simulink model "IEEE9_case"  (R2024b)
settings: Solver=FixedStepAuto  StartTime=0  StopTime=5  FixedStep=1e-7  RelTol=1e-3
values from neighbouring files (symbols this model uses):
  SG_D_1_D = 0.01056    [IEEE9_case_parameters.m]    (also in case1_parameters.m; case2_parameters.m; case3_parameters.m; case4_parameters.m)
  SG_D_1_EnableSaturation = 0    [IEEE9_case_parameters.m]    (also in case1_parameters.m; case2_parameters.m; case3_parameters.m; case4_parameters.m)
  SG_D_1_f0 = 60    [IEEE9_case_parameters.m]    (also in case1_parameters.m; case2_parameters.m; case3_parameters.m; case4_parameters.m)
  SG_D_1_H = 7.5    [IEEE9_case_parameters.m]    (also in case1_parameters.m; case2_parameters.m; case3_parameters.m; case4_parameters.m)
  SG_D_1_K_A = 20    [IEEE9_case_parameters.m]    (also in case1_parameters.m; case2_parameters.m; case3_parameters.m; case4_parameters.m)
  SG_D_1_K_E = 1.000000e+1    (= 10)    [IEEE9_case_parameters.m]    (also in case1_parameters.m; case2_parameters.m; case3_parameters.m; case4_parameters.m)
  SG_D_1_K_F = 2.363    [IEEE9_case_parameters.m]    (also in case1_parameters.m; case2_parameters.m; case3_parameters.m; case4_parameters.m)
  SG_D_1_K_s = 0.5    [IEEE9_case_parameters.m]    (also in case1_parameters.m = 5; case2_parameters.m = 5; case3_parameters.m = 5; case4_parameters.m = 5)
  SG_D_1_R_a = 0.001088    [IEEE9_case_parameters.m]    (also in case1_parameters.m; case2_parameters.m; case3_parameters.m; case4_parameters.m)
  SG_D_1_S_A = 1    [IEEE9_case_parameters.m]    (also in case1_parameters.m; case2_parameters.m; case3_parameters.m; case4_parameters.m)
  SG_D_1_S_B = 0.103    [IEEE9_case_parameters.m]    (also in case1_parameters.m; case2_parameters.m; case3_parameters.m; case4_parameters.m)
  SG_D_1_S_N = 10.659857    [IEEE9_case_parameters.m]    (also in case1_parameters.m; case2_parameters.m; case3_parameters.m; case4_parameters.m)
  SG_D_1_SpeedPara = 200    [IEEE9_case_parameters.m]    (also in case1_parameters.m; case2_parameters.m; case3_parameters.m; case4_parameters.m)
  SG_D_1_T_0 = 0.720173    [IEEE9_case_parameters.m]    (also in case1_parameters.m = 0.755522; case2_parameters.m = 0.808931; case3_parameters.m = 0.869402; case4_parameters.m = 0.729316)
  SG_D_1_T_1 = 0.3    [IEEE9_case_parameters.m]    (also in case1_parameters.m; case2_parameters.m; case3_parameters.m; case4_parameters.m)
  SG_D_1_T_2 = 0.05    [IEEE9_case_parameters.m]    (also in case1_parameters.m; case2_parameters.m; case3_parameters.m; case4_parameters.m)
  SG_D_1_T_3 = 0.02    [IEEE9_case_parameters.m]    (also in case1_parameters.m; case2_parameters.m; case3_parameters.m; case4_parameters.m)
  SG_D_1_T_4 = 0.005    [IEEE9_case_parameters.m]    (also in case1_parameters.m; case2_parameters.m; case3_parameters.m; case4_parameters.m)
  SG_D_1_T_A = 0.02    [IEEE9_case_parameters.m]    (also in case1_parameters.m; case2_parameters.m; case3_parameters.m; case4_parameters.m)
  SG_D_1_T_dd = 8.000000e+0    (= 8)    [IEEE9_case_parameters.m]    (also in case1_parameters.m; case2_parameters.m; case3_parameters.m; case4_parameters.m)
  SG_D_1_T_ddd = 0.04    [IEEE9_case_parameters.m]    (also in case1_parameters.m; case2_parameters.m; case3_parameters.m; case4_parameters.m)
  SG_D_1_T_E = 0.314    [IEEE9_case_parameters.m]    (also in case1_parameters.m; case2_parameters.m; case3_parameters.m; case4_parameters.m)
  SG_D_1_T_F = 0.35    [IEEE9_case_parameters.m]    (also in case1_parameters.m; case2_parameters.m; case3_parameters.m; case4_parameters.m)
  SG_D_1_T_qd = 0.8    [IEEE9_case_parameters.m]    (also in case1_parameters.m; case2_parameters.m; case3_parameters.m; case4_parameters.m)
  SG_D_1_T_qdd = 0.02    [IEEE9_case_parameters.m]    (also in case1_parameters.m; case2_parameters.m; case3_parameters.m; case4_parameters.m)
  SG_D_1_T_speed = 0.1    [IEEE9_case_parameters.m]    (also in case1_parameters.m = 200; case2_parameters.m = 200; case3_parameters.m = 200; case4_parameters.m = 200)
  SG_D_1_T_w = 0.5    [IEEE9_case_parameters.m]    (also in case1_parameters.m; case2_parameters.m; case3_parameters.m; case4_parameters.m)
  SG_D_1_V_ref = 1.990276    [IEEE9_case_parameters.m]    (also in case1_parameters.m = 2.042296; case2_parameters.m = 2.051388; case3_parameters.m = 2.089584; case4_parameters.m = 2.01845)
  SG_D_1_w_ref = 376.991118    [IEEE9_case_parameters.m]    (also in case1_parameters.m; case2_parameters.m; case3_parameters.m; case4_parameters.m)
  SG_D_1_wb = 6.000000e+1    (= 60)    [IEEE9_case_parameters.m]    (also in case1_parameters.m; case2_parameters.m; case3_parameters.m; case4_parameters.m)
  SG_D_1_x_d = 1.9    [IEEE9_case_parameters.m]    (also in case1_parameters.m; case2_parameters.m; case3_parameters.m; case4_parameters.m)
  SG_D_1_x_dd = 0.302    [IEEE9_case_parameters.m]    (also in case1_parameters.m; case2_parameters.m; case3_parameters.m; case4_parameters.m)
  SG_D_1_x_ddd = 0.204    [IEEE9_case_parameters.m]    (also in case1_parameters.m; case2_parameters.m; case3_parameters.m; case4_parameters.m)
  SG_D_1_x_l = 0.05    [IEEE9_case_parameters.m]    (also in case1_parameters.m; case2_parameters.m; case3_parameters.m; case4_parameters.m)
  SG_D_1_x_q = 1.3    [IEEE9_case_parameters.m]    (also in case1_parameters.m; case2_parameters.m; case3_parameters.m; case4_parameters.m)
  SG_D_1_x_qd = 0.5    [IEEE9_case_parameters.m]    (also in case1_parameters.m; case2_parameters.m; case3_parameters.m; case4_parameters.m)
  SG_D_1_x_qdd = 0.3    [IEEE9_case_parameters.m]    (also in case1_parameters.m; case2_parameters.m; case3_parameters.m; case4_parameters.m)
  SG_D_2_D = 0.02    [IEEE9_case_parameters.m]    (also in case1_parameters.m; case2_parameters.m; case3_parameters.m; case4_parameters.m)
  SG_D_2_EnableSaturation = 0    [IEEE9_case_parameters.m]    (also in case1_parameters.m; case2_parameters.m; case3_parameters.m; case4_parameters.m)
  SG_D_2_f0 = 60    [IEEE9_case_parameters.m]    (also in case1_parameters.m; case2_parameters.m; case3_parameters.m; case4_parameters.m)
  SG_D_2_H = 8.000000e+0    (= 8)    [IEEE9_case_parameters.m]    (also in case1_parameters.m; case2_parameters.m; case3_parameters.m; case4_parameters.m)
  SG_D_2_K_A = 20    [IEEE9_case_parameters.m]    (also in case1_parameters.m; case2_parameters.m; case3_parameters.m; case4_parameters.m)
  SG_D_2_K_E = 1.000000e+1    (= 10)    [IEEE9_case_parameters.m]    (also in case1_parameters.m; case2_parameters.m; case3_parameters.m; case4_parameters.m)
  SG_D_2_K_F = 2.363    [IEEE9_case_parameters.m]    (also in case1_parameters.m; case2_parameters.m; case3_parameters.m; case4_parameters.m)
  SG_D_2_K_s = 0.5    [IEEE9_case_parameters.m]    (also in case1_parameters.m = 4; case2_parameters.m = 4; case3_parameters.m = 4; case4_parameters.m = 4)
  SG_D_2_R_a = 0.001088    [IEEE9_case_parameters.m]    (also in case1_parameters.m; case2_parameters.m; case3_parameters.m; case4_parameters.m)
  SG_D_2_S_A = 1    [IEEE9_case_parameters.m]    (also in case1_parameters.m; case2_parameters.m; case3_parameters.m; case4_parameters.m)
  SG_D_2_S_B = 0.103    [IEEE9_case_parameters.m]    (also in case1_parameters.m; case2_parameters.m; case3_parameters.m; case4_parameters.m)
  SG_D_2_S_N = 10.659857    [IEEE9_case_parameters.m]    (also in case1_parameters.m; case2_parameters.m; case3_parameters.m; case4_parameters.m)
  SG_D_2_SpeedPara = 200    [IEEE9_case_parameters.m]    (also in case1_parameters.m; case2_parameters.m; case3_parameters.m; case4_parameters.m)
  SG_D_2_T_0 = 1.632913    [IEEE9_case_parameters.m]    (also in case1_parameters.m = 1.632925; case2_parameters.m = 1.632915; case3_parameters.m = 1.632914; case4_parameters.m = 1.632927)
  SG_D_2_T_1 = 0.2    [IEEE9_case_parameters.m]    (also in case1_parameters.m; case2_parameters.m; case3_parameters.m; case4_parameters.m)
  SG_D_2_T_2 = 0.05    [IEEE9_case_parameters.m]    (also in case1_parameters.m; case2_parameters.m; case3_parameters.m; case4_parameters.m)
  SG_D_2_T_3 = 0.02    [IEEE9_case_parameters.m]    (also in case1_parameters.m; case2_parameters.m; case3_parameters.m; case4_parameters.m)
  SG_D_2_T_4 = 0.005    [IEEE9_case_parameters.m]    (also in case1_parameters.m; case2_parameters.m; case3_parameters.m; case4_parameters.m)
  SG_D_2_T_A = 0.02    [IEEE9_case_parameters.m]    (also in case1_parameters.m; case2_parameters.m; case3_parameters.m; case4_parameters.m)
  SG_D_2_T_dd = 7.9    [IEEE9_case_parameters.m]    (also in case1_parameters.m; case2_parameters.m; case3_parameters.m; case4_parameters.m)
  SG_D_2_T_ddd = 0.04    [IEEE9_case_parameters.m]    (also in case1_parameters.m; case2_parameters.m; case3_parameters.m; case4_parameters.m)
  SG_D_2_T_E = 0.314    [IEEE9_case_parameters.m]    (also in case1_parameters.m; case2_parameters.m; case3_parameters.m; case4_parameters.m)
  SG_D_2_T_F = 0.35    [IEEE9_case_parameters.m]    (also in case1_parameters.m; case2_parameters.m; case3_parameters.m; case4_parameters.m)
  SG_D_2_T_qd = 0.8    [IEEE9_case_parameters.m]    (also in case1_parameters.m; case2_parameters.m; case3_parameters.m; case4_parameters.m)
  SG_D_2_T_qdd = 0.015    [IEEE9_case_parameters.m]    (also in case1_parameters.m; case2_parameters.m; case3_parameters.m; case4_parameters.m)
  SG_D_2_T_speed = 0.1    [IEEE9_case_parameters.m]    (also in case1_parameters.m = 150; case2_parameters.m = 150; case3_parameters.m = 150; case4_parameters.m = 150)
  SG_D_2_T_w = 0.35    [IEEE9_case_parameters.m]    (also in case1_parameters.m; case2_parameters.m; case3_parameters.m; case4_parameters.m)
  SG_D_2_V_ref = 2.58547    [IEEE9_case_parameters.m]    (also in case1_parameters.m = 2.597896; case2_parameters.m = 2.587136; case3_parameters.m = 2.586042; case4_parameters.m = 2.599679)
  SG_D_2_w_ref = 376.991118    [IEEE9_case_parameters.m]    (also in case1_parameters.m; case2_parameters.m; case3_parameters.m; case4_parameters.m)
  SG_D_2_wb = 6.000000e+1    (= 60)    [IEEE9_case_parameters.m]    (also in case1_parameters.m; case2_parameters.m; case3_parameters.m; case4_parameters.m)
  SG_D_2_x_d = 1.8    [IEEE9_case_parameters.m]    (also in case1_parameters.m; case2_parameters.m; case3_parameters.m; case4_parameters.m)
  SG_D_2_x_dd = 0.302    [IEEE9_case_parameters.m]    (also in case1_parameters.m; case2_parameters.m; case3_parameters.m; case4_parameters.m)
  SG_D_2_x_ddd = 0.204    [IEEE9_case_parameters.m]    (also in case1_parameters.m; case2_parameters.m; case3_parameters.m; case4_parameters.m)
  SG_D_2_x_l = 0.05    [IEEE9_case_parameters.m]    (also in case1_parameters.m; case2_parameters.m; case3_parameters.m; case4_parameters.m)
  SG_D_2_x_q = 1.25    [IEEE9_case_parameters.m]    (also in case1_parameters.m; case2_parameters.m; case3_parameters.m; case4_parameters.m)
  SG_D_2_x_qd = 0.5    [IEEE9_case_parameters.m]    (also in case1_parameters.m; case2_parameters.m; case3_parameters.m; case4_parameters.m)
  SG_D_2_x_qdd = 0.3    [IEEE9_case_parameters.m]    (also in case1_parameters.m; case2_parameters.m; case3_parameters.m; case4_parameters.m)
  SG_D_3_D = 0.02    [IEEE9_case_parameters.m]    (also in case1_parameters.m; case2_parameters.m; case3_parameters.m; case4_parameters.m)
  SG_D_3_EnableSaturation = 0    [IEEE9_case_parameters.m]    (also in case1_parameters.m; case2_parameters.m; case3_parameters.m; case4_parameters.m)
  SG_D_3_f0 = 60    [IEEE9_case_parameters.m]    (also in case1_parameters.m; case2_parameters.m; case3_parameters.m; case4_parameters.m)
  SG_D_3_H = 7.7    [IEEE9_case_parameters.m]    (also in case1_parameters.m; case2_parameters.m; case3_parameters.m; case4_parameters.m)
  SG_D_3_K_A = 20    [IEEE9_case_parameters.m]    (also in case1_parameters.m; case2_parameters.m; case3_parameters.m; case4_parameters.m)
  SG_D_3_K_E = 1.000000e+1    (= 10)    [IEEE9_case_parameters.m]    (also in case1_parameters.m; case2_parameters.m; case3_parameters.m; case4_parameters.m)
  SG_D_3_K_F = 2.363    [IEEE9_case_parameters.m]    (also in case1_parameters.m; case2_parameters.m; case3_parameters.m; case4_parameters.m)
  SG_D_3_K_s = 0.2    [IEEE9_case_parameters.m]    (also in case1_parameters.m = 2; case2_parameters.m = 2; case3_parameters.m = 2; case4_parameters.m = 2)
  SG_D_3_R_a = 0.001088    [IEEE9_case_parameters.m]    (also in case1_parameters.m; case2_parameters.m; case3_parameters.m; case4_parameters.m)
  SG_D_3_S_A = 1    [IEEE9_case_parameters.m]    (also in case1_parameters.m; case2_parameters.m; case3_parameters.m; case4_parameters.m)
  SG_D_3_S_B = 0.103    [IEEE9_case_parameters.m]    (also in case1_parameters.m; case2_parameters.m; case3_parameters.m; case4_parameters.m)
  SG_D_3_S_N = 10.659857    [IEEE9_case_parameters.m]    (also in case1_parameters.m; case2_parameters.m; case3_parameters.m; case4_parameters.m)
  SG_D_3_SpeedPara = 200    [IEEE9_case_parameters.m]    (also in case1_parameters.m; case2_parameters.m; case3_parameters.m; case4_parameters.m)
  SG_D_3_T_0 = 0.850788    [IEEE9_case_parameters.m]    (also in case1_parameters.m = 0.850786; case2_parameters.m = 0.850787; case3_parameters.m; case4_parameters.m = 0.850786)
  SG_D_3_T_1 = 0.2    [IEEE9_case_parameters.m]    (also in case1_parameters.m; case2_parameters.m; case3_parameters.m; case4_parameters.m)
  SG_D_3_T_2 = 0.05    [IEEE9_case_parameters.m]    (also in case1_parameters.m; case2_parameters.m; case3_parameters.m; case4_parameters.m)
  SG_D_3_T_3 = 0.02    [IEEE9_case_parameters.m]    (also in case1_parameters.m; case2_parameters.m; case3_parameters.m; case4_parameters.m)
  SG_D_3_T_4 = 0.005    [IEEE9_case_parameters.m]    (also in case1_parameters.m; case2_parameters.m; case3_parameters.m; case4_parameters.m)
  SG_D_3_T_A = 0.02    [IEEE9_case_parameters.m]    (also in case1_parameters.m; case2_parameters.m; case3_parameters.m; case4_parameters.m)
  SG_D_3_T_dd = 8.1    [IEEE9_case_parameters.m]    (also in case1_parameters.m; case2_parameters.m; case3_parameters.m; case4_parameters.m)
  SG_D_3_T_ddd = 0.04    [IEEE9_case_parameters.m]    (also in case1_parameters.m; case2_parameters.m; case3_parameters.m; case4_parameters.m)
  SG_D_3_T_E = 0.314    [IEEE9_case_parameters.m]    (also in case1_parameters.m; case2_parameters.m; case3_parameters.m; case4_parameters.m)
  SG_D_3_T_F = 0.35    [IEEE9_case_parameters.m]    (also in case1_parameters.m; case2_parameters.m; case3_parameters.m; case4_parameters.m)
  SG_D_3_T_qd = 0.8    [IEEE9_case_parameters.m]    (also in case1_parameters.m; case2_parameters.m; case3_parameters.m; case4_parameters.m)
  SG_D_3_T_qdd = 0.015    [IEEE9_case_parameters.m]    (also in case1_parameters.m; case2_parameters.m; case3_parameters.m; case4_parameters.m)
  SG_D_3_T_speed = 0.1    [IEEE9_case_parameters.m]    (also in case1_parameters.m = 180; case2_parameters.m = 180; case3_parameters.m = 180; case4_parameters.m = 180)
  SG_D_3_T_w = 0.4    [IEEE9_case_parameters.m]    (also in case1_parameters.m; case2_parameters.m; case3_parameters.m; case4_parameters.m)
  SG_D_3_V_ref = 1.892727    [IEEE9_case_parameters.m]    (also in case1_parameters.m = 1.906439; case2_parameters.m = 1.895535; case3_parameters.m = 1.892105; case4_parameters.m = 1.906598)
  SG_D_3_w_ref = 376.991118    [IEEE9_case_parameters.m]    (also in case1_parameters.m; case2_parameters.m; case3_parameters.m; case4_parameters.m)
  SG_D_3_wb = 6.000000e+1    (= 60)    [IEEE9_case_parameters.m]    (also in case1_parameters.m; case2_parameters.m; case3_parameters.m; case4_parameters.m)
  SG_D_3_x_d = 1.85    [IEEE9_case_parameters.m]    (also in case1_parameters.m; case2_parameters.m; case3_parameters.m; case4_parameters.m)
  SG_D_3_x_dd = 0.302    [IEEE9_case_parameters.m]    (also in case1_parameters.m; case2_parameters.m; case3_parameters.m; case4_parameters.m)
  SG_D_3_x_ddd = 0.204    [IEEE9_case_parameters.m]    (also in case1_parameters.m; case2_parameters.m; case3_parameters.m; case4_parameters.m)
  SG_D_3_x_l = 0.05    [IEEE9_case_parameters.m]    (also in case1_parameters.m; case2_parameters.m; case3_parameters.m; case4_parameters.m)
  SG_D_3_x_q = 1.2    [IEEE9_case_parameters.m]    (also in case1_parameters.m; case2_parameters.m; case3_parameters.m; case4_parameters.m)
  SG_D_3_x_qd = 0.5    [IEEE9_case_parameters.m]    (also in case1_parameters.m; case2_parameters.m; case3_parameters.m; case4_parameters.m)
  SG_D_3_x_qdd = 0.3    [IEEE9_case_parameters.m]    (also in case1_parameters.m; case2_parameters.m; case3_parameters.m; case4_parameters.m)
(part 3 of 12)

== system IEEE9_case/AC_1/d_id_line_9_4_block ==
  note: d_id_line_9_4 in IEEE9_case
      | $376.991118430775\,\mathrm{iq}_{\mathrm{line},9,4}-44.3518962859735\,\mathrm{id}_{\mathrm{line},9,4}-4435.18962859735\,\mathrm{vd}_{\mathrm{bus},4}+4435.18962859735\,\mathrm{vd}_{\mathrm{bus},9}$
      | Automatically generated on 2025-11-01 08:51:15 .
  State_id_line_9_4_4873b : Inport
  State_iq_line_9_4_6aab9 : Inport  Port=2
  State_vd_bus_4_38073 : Inport  Port=3
  State_vd_bus_9_760c0 : Inport  Port=4
  Add_56f63 : Sum
  Add_c2ec8 : Sum
  Constant_-44.3518962859735_f091e : Constant  Value=-44.3518962859735
  Constant_376.991118430775_dc17f : Constant  Value=376.991118430775
  Constant_4435.18962859735_86132 : Constant  Value=4435.18962859735
  Constant_4435.18962859735_9a60c : Constant  Value=4435.18962859735
  Product_6f2af : Product
  Product_a8ea4 : Product
  Product_bd232 : Product
  Product_c2f22 : Product
  Subtract_43f53 : Sum  Inputs=+-
  Blockout_d_id_line_9_4_80f4f : Outport
  wires:
  Constant_-44.3518962859735_f091e/1 -> Product_6f2af/1
  Product_bd232/1 -> Add_c2ec8/2
  State_id_line_9_4_4873b/1 -> Product_6f2af/2
  Constant_376.991118430775_dc17f/1 -> Product_bd232/1
  Product_6f2af/1 -> Add_c2ec8/1
  State_iq_line_9_4_6aab9/1 -> Product_bd232/2
  Constant_4435.18962859735_86132/1 -> Product_c2f22/1
  State_vd_bus_4_38073/1 -> Product_c2f22/2
  Add_c2ec8/1 -> Subtract_43f53/1
  Product_c2f22/1 -> Subtract_43f53/2
  Constant_4435.18962859735_9a60c/1 -> Product_a8ea4/1
  Subtract_43f53/1 -> Add_56f63/1
  State_vd_bus_9_760c0/1 -> Product_a8ea4/2
  Product_a8ea4/1 -> Add_56f63/2
  Add_56f63/1 -> Blockout_d_id_line_9_4_80f4f/1

== system IEEE9_case/AC_1/d_id_load_5_block ==
  note: d_id_load_5 in IEEE9_case
      | $376.991118430775\,\mathrm{iq}_{\mathrm{load},5}-1130.97335529233\,\mathrm{id}_{\mathrm{load},5}+1188.5640696821\,\mathrm{vd}_{\mathrm{bus},5}$
      | Automatically generated on 2025-11-01 08:50:52 .
  State_id_load_5_2b1bb : Inport
  State_iq_load_5_ef704 : Inport  Port=2
  State_vd_bus_5_2ec2f : Inport  Port=3
  Add_0c269 : Sum
  Add_56efd : Sum
  Constant_-1130.97335529233_ef54c : Constant  Value=-1130.97335529233
  Constant_1188.5640696821_c8414 : Constant  Value=1188.5640696821
  Constant_376.991118430775_cc731 : Constant  Value=376.991118430775
  Product_9d4ce : Product
  Product_ba4c9 : Product
  Product_dacee : Product
  Blockout_d_id_load_5_45067 : Outport
  wires:
  Constant_-1130.97335529233_ef54c/1 -> Product_ba4c9/1
  Product_dacee/1 -> Add_0c269/2
  State_id_load_5_2b1bb/1 -> Product_ba4c9/2
  Constant_376.991118430775_cc731/1 -> Product_dacee/1
  Product_9d4ce/1 -> Add_56efd/2
  State_iq_load_5_ef704/1 -> Product_dacee/2
  Product_ba4c9/1 -> Add_0c269/1
  Constant_1188.5640696821_c8414/1 -> Product_9d4ce/1
  State_vd_bus_5_2ec2f/1 -> Product_9d4ce/2
  Add_0c269/1 -> Add_56efd/1
  Add_56efd/1 -> Blockout_d_id_load_5_45067/1

== system IEEE9_case/AC_1/d_id_load_7_block ==
  note: d_id_load_7 in IEEE9_case
      | $376.991118430775\,\mathrm{iq}_{\mathrm{load},7}-1077.11748123079\,\mathrm{id}_{\mathrm{load},7}+1244.53892235533\,\mathrm{vd}_{\mathrm{bus},7}$
      | Automatically generated on 2025-11-01 08:50:54 .
  State_id_load_7_85756 : Inport
  State_iq_load_7_0d377 : Inport  Port=2
  State_vd_bus_7_4e44c : Inport  Port=3
  Add_67116 : Sum
  Add_7cb0d : Sum
  Constant_-1077.11748123079_6ed19 : Constant  Value=-1077.11748123079
  Constant_1244.53892235533_2ed2b : Constant  Value=1244.53892235533
  Constant_376.991118430775_5e070 : Constant  Value=376.991118430775
  Product_90d80 : Product
  Product_aba60 : Product
  Product_bc1cf : Product
  Blockout_d_id_load_7_0150f : Outport
  wires:
  Constant_-1077.11748123079_6ed19/1 -> Product_bc1cf/1
  Product_aba60/1 -> Add_7cb0d/2
  State_id_load_7_85756/1 -> Product_bc1cf/2
  Constant_376.991118430775_5e070/1 -> Product_aba60/1
  Product_bc1cf/1 -> Add_7cb0d/1
  State_iq_load_7_0d377/1 -> Product_aba60/2
  Constant_1244.53892235533_2ed2b/1 -> Product_90d80/1
  State_vd_bus_7_4e44c/1 -> Product_90d80/2
  Add_7cb0d/1 -> Add_67116/1
  Product_90d80/1 -> Add_67116/2
  Add_67116/1 -> Blockout_d_id_load_7_0150f/1

== system IEEE9_case/AC_1/d_id_load_9_block ==
  note: d_id_load_9 in IEEE9_case
      | $376.991118430775\,\mathrm{iq}_{\mathrm{load},9}-942.477796076938\,\mathrm{id}_{\mathrm{load},9}+1490.22474585066\,\mathrm{vd}_{\mathrm{bus},9}$
      | Automatically generated on 2025-11-01 08:50:56 .
  State_id_load_9_adb15 : Inport
  State_iq_load_9_1d7e2 : Inport  Port=2
  State_vd_bus_9_f7f95 : Inport  Port=3
  Add_7caa6 : Sum
  Add_fe44a : Sum
  Constant_-942.477796076938_470ff : Constant  Value=-942.477796076938
  Constant_1490.22474585066_bf519 : Constant  Value=1490.22474585066
  Constant_376.991118430775_83929 : Constant  Value=376.991118430775
  Product_37c77 : Product
  Product_62471 : Product
  Product_a02c9 : Product
  Blockout_d_id_load_9_c2cf2 : Outport
  wires:
  Constant_-942.477796076938_470ff/1 -> Product_a02c9/1
  Product_62471/1 -> Add_fe44a/2
  State_id_load_9_adb15/1 -> Product_a02c9/2
  Constant_376.991118430775_83929/1 -> Product_62471/1
  Product_a02c9/1 -> Add_fe44a/1
  State_iq_load_9_1d7e2/1 -> Product_62471/2
  Constant_1490.22474585066_bf519/1 -> Product_37c77/1
  State_vd_bus_9_f7f95/1 -> Product_37c77/2
  Add_fe44a/1 -> Add_7caa6/1
  Product_37c77/1 -> Add_7caa6/2
  Add_7caa6/1 -> Blockout_d_id_load_9_c2cf2/1

== system IEEE9_case/AC_1/d_iq_line_1_4_block ==
  note: d_iq_line_1_4 in IEEE9_case
      | $6544.98469497874\,\mathrm{vq}_{\mathrm{bus},1}-376.991118430775\,\mathrm{id}_{\mathrm{line},1,4}-6544.98469497874\,\mathrm{vq}_{\mathrm{bus},4}$
      | Automatically generated on 2025-11-01 08:50:59 .
  State_id_line_1_4_423c5 : Inport
  State_vq_bus_1_85cee : Inport  Port=2
  State_vq_bus_4_61231 : Inport  Port=3
  Add_ad111 : Sum
  Constant_-376.991118430775_35d49 : Constant  Value=-376.991118430775
  Constant_6544.98469497874_957e0 : Constant  Value=6544.98469497874
  Constant_6544.98469497874_e68d1 : Constant  Value=6544.98469497874
  Product_2a856 : Product
  Product_35aa0 : Product
  Product_cca18 : Product
  Subtract_8cf3b : Sum  Inputs=+-
  Blockout_d_iq_line_1_4_8e08d : Outport
  wires:
  Constant_-376.991118430775_35d49/1 -> Product_2a856/1
  Product_35aa0/1 -> Add_ad111/2
  State_id_line_1_4_423c5/1 -> Product_2a856/2
  Constant_6544.98469497874_e68d1/1 -> Product_35aa0/1
  Product_2a856/1 -> Add_ad111/1
  Subtract_8cf3b/1 -> Blockout_d_iq_line_1_4_8e08d/1
  State_vq_bus_1_85cee/1 -> Product_35aa0/2
  Constant_6544.98469497874_957e0/1 -> Product_cca18/1
  State_vq_bus_4_61231/1 -> Product_cca18/2
  Add_ad111/1 -> Subtract_8cf3b/1
  Product_cca18/1 -> Subtract_8cf3b/2

== system IEEE9_case/AC_1/d_iq_line_3_6_block ==
  note: d_iq_line_3_6 in IEEE9_case
      | $6433.29553636135\,\mathrm{vq}_{\mathrm{bus},3}-376.991118430775\,\mathrm{id}_{\mathrm{line},3,6}-6433.29553636135\,\mathrm{vq}_{\mathrm{bus},6}$
      | Automatically generated on 2025-11-01 08:51:05 .
  State_id_line_3_6_009c9 : Inport
  State_vq_bus_3_bedda : Inport  Port=2
  State_vq_bus_6_3dee8 : Inport  Port=3
  Add_35b3d : Sum
  Constant_-376.991118430775_7363e : Constant  Value=-376.991118430775
  Constant_6433.29553636135_1c8cb : Constant  Value=6433.29553636135
  Constant_6433.29553636135_28456 : Constant  Value=6433.29553636135
  Product_50921 : Product
  Product_53ffc : Product
  Product_6f551 : Product
  Subtract_0e2f7 : Sum  Inputs=+-
  Blockout_d_iq_line_3_6_efa2c : Outport
  wires:
  Constant_-376.991118430775_7363e/1 -> Product_50921/1
  Product_6f551/1 -> Add_35b3d/2
  State_id_line_3_6_009c9/1 -> Product_50921/2
  Constant_6433.29553636135_1c8cb/1 -> Product_6f551/1
  Product_50921/1 -> Add_35b3d/1
  State_vq_bus_3_bedda/1 -> Product_6f551/2
  Constant_6433.29553636135_28456/1 -> Product_53ffc/1
  State_vq_bus_6_3dee8/1 -> Product_53ffc/2
  Add_35b3d/1 -> Subtract_0e2f7/1
  Product_53ffc/1 -> Subtract_0e2f7/2
  Subtract_0e2f7/1 -> Blockout_d_iq_line_3_6_efa2c/1

== system IEEE9_case/AC_1/d_iq_line_4_5_block ==
  note: d_iq_line_4_5 in IEEE9_case
      | $4097.7295481606\,\mathrm{vq}_{\mathrm{bus},4}-69.6614023187302\,\mathrm{iq}_{\mathrm{line},4,5}-376.991118430775\,\mathrm{id}_{\mathrm{line},4,5}-4097.7295481606\,\mathrm{vq}_{\mathrm{bus},5}$
      | Automatically generated on 2025-11-01 08:51:01 .
  State_id_line_4_5_3365c : Inport
  State_iq_line_4_5_213cd : Inport  Port=2
  State_vq_bus_4_01a8c : Inport  Port=3
  State_vq_bus_5_00127 : Inport  Port=4
  Add_6421a : Sum
  Constant_-376.991118430775_1a696 : Constant  Value=-376.991118430775
  Constant_4097.7295481606_9b4f7 : Constant  Value=4097.7295481606
  Constant_4097.7295481606_ed17d : Constant  Value=4097.7295481606
  Constant_69.6614023187302_4ac1b : Constant  Value=69.6614023187302
  Product_1e8b7 : Product
  Product_40df5 : Product
  Product_75e53 : Product
  Product_bf0ee : Product
  Subtract_31b75 : Sum  Inputs=+-
  Subtract_9f617 : Sum  Inputs=+-
  Blockout_d_iq_line_4_5_f1556 : Outport
  wires:
  Constant_-376.991118430775_1a696/1 -> Product_bf0ee/1
  Constant_69.6614023187302_4ac1b/1 -> Product_1e8b7/1
  State_id_line_4_5_3365c/1 -> Product_bf0ee/2
  State_iq_line_4_5_213cd/1 -> Product_1e8b7/2
  Product_bf0ee/1 -> Subtract_31b75/1
  Constant_4097.7295481606_9b4f7/1 -> Product_75e53/1
  Product_1e8b7/1 -> Subtract_31b75/2
  State_vq_bus_4_01a8c/1 -> Product_75e53/2
  Subtract_31b75/1 -> Add_6421a/1
  Product_75e53/1 -> Add_6421a/2
  Constant_4097.7295481606_ed17d/1 -> Product_40df5/1
  State_vq_bus_5_00127/1 -> Product_40df5/2
  Add_6421a/1 -> Subtract_9f617/1
  Product_40df5/1 -> Subtract_9f617/2
  Subtract_9f617/1 -> Blockout_d_iq_line_4_5_f1556/1

== system IEEE9_case/AC_1/d_iq_line_5_6_block ==
  note: d_iq_line_5_6 in IEEE9_case
      | $2217.59481429868\,\mathrm{vq}_{\mathrm{bus},5}-86.4861977576484\,\mathrm{iq}_{\mathrm{line},5,6}-376.991118430775\,\mathrm{id}_{\mathrm{line},5,6}-2217.59481429868\,\mathrm{vq}_{\mathrm{bus},6}$
      | Automatically generated on 2025-11-01 08:51:03 .
  State_id_line_5_6_c9e53 : Inport
  State_iq_line_5_6_c9448 : Inport  Port=2
  State_vq_bus_5_5d45c : Inport  Port=3
  State_vq_bus_6_316f0 : Inport  Port=4
  Add_651ea : Sum
  Constant_-376.991118430775_76bfa : Constant  Value=-376.991118430775
  Constant_2217.59481429868_82eaa : Constant  Value=2217.59481429868
  Constant_2217.59481429868_9c552 : Constant  Value=2217.59481429868
  Constant_86.4861977576484_c0996 : Constant  Value=86.4861977576484
  Product_5487f : Product
  Product_62c6c : Product
  Product_8b71f : Product
  Product_c3fc5 : Product
  Subtract_7da67 : Sum  Inputs=+-
  Subtract_ad5d5 : Sum  Inputs=+-
  Blockout_d_iq_line_5_6_dbe92 : Outport
  wires:
  Constant_-376.991118430775_76bfa/1 -> Product_c3fc5/1
  Constant_86.4861977576484_c0996/1 -> Product_8b71f/1
  Subtract_7da67/1 -> Blockout_d_iq_line_5_6_dbe92/1
  State_id_line_5_6_c9e53/1 -> Product_c3fc5/2
  State_iq_line_5_6_c9448/1 -> Product_8b71f/2
  Product_c3fc5/1 -> Subtract_ad5d5/1
  Constant_2217.59481429868_9c552/1 -> Product_62c6c/1
  Product_8b71f/1 -> Subtract_ad5d5/2
  Product_5487f/1 -> Subtract_7da67/2
  State_vq_bus_5_5d45c/1 -> Product_62c6c/2
  Subtract_ad5d5/1 -> Add_651ea/1
  Product_62c6c/1 -> Add_651ea/2
  Constant_2217.59481429868_82eaa/1 -> Product_5487f/1
  State_vq_bus_6_316f0/1 -> Product_5487f/2
  Add_651ea/1 -> Subtract_7da67/1

== system IEEE9_case/AC_1/d_iq_line_6_7_block ==
  note: d_iq_line_6_7 in IEEE9_case
      | $3739.99125427356\,\mathrm{vq}_{\mathrm{bus},6}-44.5058959258554\,\mathrm{iq}_{\mathrm{line},6,7}-376.991118430775\,\mathrm{id}_{\mathrm{line},6,7}-3739.99125427356\,\mathrm{vq}_{\mathrm{bus},7}$
      | Automatically generated on 2025-11-01 08:51:08 .
  State_id_line_6_7_f8f8d : Inport
  State_iq_line_6_7_dab1d : Inport  Port=2
  State_vq_bus_6_46bfc : Inport  Port=3
  State_vq_bus_7_7f00d : Inport  Port=4
  Add_cb784 : Sum
  Constant_-376.991118430775_4ea49 : Constant  Value=-376.991118430775
  Constant_3739.99125427356_4ae0d : Constant  Value=3739.99125427356
  Constant_3739.99125427356_7f880 : Constant  Value=3739.99125427356
  Constant_44.5058959258554_6a478 : Constant  Value=44.5058959258554
  Product_45817 : Product
  Product_62dbb : Product
  Product_d7e7b : Product
  Product_ebd48 : Product
  Subtract_13366 : Sum  Inputs=+-
  Subtract_b174f : Sum  Inputs=+-
  Blockout_d_iq_line_6_7_dacae : Outport
  wires:
  Constant_-376.991118430775_4ea49/1 -> Product_62dbb/1
  Constant_44.5058959258554_6a478/1 -> Product_ebd48/1
  State_id_line_6_7_f8f8d/1 -> Product_62dbb/2
  State_iq_line_6_7_dab1d/1 -> Product_ebd48/2
  Product_62dbb/1 -> Subtract_b174f/1
  Constant_3739.99125427356_7f880/1 -> Product_45817/1
  Product_ebd48/1 -> Subtract_b174f/2
  State_vq_bus_6_46bfc/1 -> Product_45817/2
  Subtract_b174f/1 -> Add_cb784/1
  Product_45817/1 -> Add_cb784/2
  Constant_3739.99125427356_4ae0d/1 -> Product_d7e7b/1
  State_vq_bus_7_7f00d/1 -> Product_d7e7b/2
  Add_cb784/1 -> Subtract_13366/1
  Product_d7e7b/1 -> Subtract_13366/2
  Subtract_13366/1 -> Blockout_d_iq_line_6_7_dacae/1

== system IEEE9_case/AC_1/d_iq_line_7_8_block ==
  note: d_iq_line_7_8 in IEEE9_case
      | $5235.98775598299\,\mathrm{vq}_{\mathrm{bus},7}-44.5058959258554\,\mathrm{iq}_{\mathrm{line},7,8}-376.991118430775\,\mathrm{id}_{\mathrm{line},7,8}-5235.98775598299\,\mathrm{vq}_{\mathrm{bus},8}$
      | Automatically generated on 2025-11-01 08:51:10 .
  State_id_line_7_8_c97aa : Inport
  State_iq_line_7_8_1b0e2 : Inport  Port=2
  State_vq_bus_7_6e292 : Inport  Port=3
  State_vq_bus_8_9448a : Inport  Port=4
  Add_ea538 : Sum
  Constant_-376.991118430775_f2a4d : Constant  Value=-376.991118430775
  Constant_44.5058959258554_9a8c4 : Constant  Value=44.5058959258554
  Constant_5235.98775598299_0d8b9 : Constant  Value=5235.98775598299
  Constant_5235.98775598299_57d1f : Constant  Value=5235.98775598299
  Product_3450b : Product
  Product_4947e : Product
  Product_9d0dc : Product
  Product_a96b9 : Product
  Subtract_5270b : Sum  Inputs=+-
  Subtract_c1b14 : Sum  Inputs=+-
  Blockout_d_iq_line_7_8_0db81 : Outport
  wires:
  Constant_-376.991118430775_f2a4d/1 -> Product_3450b/1
  Constant_44.5058959258554_9a8c4/1 -> Product_4947e/1
  State_id_line_7_8_c97aa/1 -> Product_3450b/2
  State_iq_line_7_8_1b0e2/1 -> Product_4947e/2
  Product_3450b/1 -> Subtract_c1b14/1
  Constant_5235.98775598299_57d1f/1 -> Product_a96b9/1
  Product_4947e/1 -> Subtract_c1b14/2
  State_vq_bus_7_6e292/1 -> Product_a96b9/2
  Subtract_c1b14/1 -> Add_ea538/1
  Product_a96b9/1 -> Add_ea538/2
  Constant_5235.98775598299_0d8b9/1 -> Product_9d0dc/1
  State_vq_bus_8_9448a/1 -> Product_9d0dc/2
  Add_ea538/1 -> Subtract_5270b/1
  Product_9d0dc/1 -> Subtract_5270b/2
  Subtract_5270b/1 -> Blockout_d_iq_line_7_8_0db81/1

== system IEEE9_case/AC_1/d_iq_line_8_2_block ==
  note: d_iq_line_8_2 in IEEE9_case
      | $6031.8578948924\,\mathrm{vq}_{\mathrm{bus},8}-6031.8578948924\,\mathrm{vq}_{\mathrm{bus},2}-376.991118430775\,\mathrm{id}_{\mathrm{line},8,2}$
      | Automatically generated on 2025-11-01 08:51:12 .
  State_id_line_8_2_6fbbf : Inport
  State_vq_bus_2_442ae : Inport  Port=2
  State_vq_bus_8_09901 : Inport  Port=3
  Add_133f8 : Sum
  Constant_-376.991118430775_63922 : Constant  Value=-376.991118430775
  Constant_6031.8578948924_94afc : Constant  Value=6031.8578948924
  Constant_6031.8578948924_bae9c : Constant  Value=6031.8578948924
  Product_6e749 : Product
  Product_7cd7e : Product
  Product_f143d : Product
  Subtract_6b886 : Sum  Inputs=+-
  Blockout_d_iq_line_8_2_35d70 : Outport
  wires:
  Constant_-376.991118430775_63922/1 -> Product_6e749/1
  Product_f143d/1 -> Subtract_6b886/2
  State_id_line_8_2_6fbbf/1 -> Product_6e749/2
  Constant_6031.8578948924_bae9c/1 -> Product_f143d/1
  Product_6e749/1 -> Subtract_6b886/1
  State_vq_bus_2_442ae/1 -> Product_f143d/2
  Constant_6031.8578948924_94afc/1 -> Product_7cd7e/1
  State_vq_bus_8_09901/1 -> Product_7cd7e/2
  Subtract_6b886/1 -> Add_133f8/1
  Product_7cd7e/1 -> Add_133f8/2
  Add_133f8/1 -> Blockout_d_iq_line_8_2_35d70/1

== system IEEE9_case/AC_1/d_iq_line_8_9_block ==
  note: d_iq_line_8_9 in IEEE9_case
      | $2341.55974180606\,\mathrm{vq}_{\mathrm{bus},8}-74.9299117377938\,\mathrm{iq}_{\mathrm{line},8,9}-376.991118430775\,\mathrm{id}_{\mathrm{line},8,9}-2341.55974180606\,\mathrm{vq}_{\mathrm{bus},9}$
      | Automatically generated on 2025-11-01 08:51:14 .
  State_id_line_8_9_6201c : Inport
  State_iq_line_8_9_3d23d : Inport  Port=2
  State_vq_bus_8_ba3ce : Inport  Port=3
  State_vq_bus_9_94e60 : Inport  Port=4
  Add_051e8 : Sum
  Constant_-376.991118430775_074d9 : Constant  Value=-376.991118430775
  Constant_2341.55974180606_2b1bb : Constant  Value=2341.55974180606
  Constant_2341.55974180606_e9be4 : Constant  Value=2341.55974180606
  Constant_74.9299117377938_59622 : Constant  Value=74.9299117377938
  Product_5be2d : Product
  Product_7e30b : Product
  Product_aa549 : Product
  Product_d55c5 : Product
  Subtract_9c8a5 : Sum  Inputs=+-
  Subtract_f6bd1 : Sum  Inputs=+-
  Blockout_d_iq_line_8_9_1ac9c : Outport
  wires:
  Constant_-376.991118430775_074d9/1 -> Product_5be2d/1
  Constant_74.9299117377938_59622/1 -> Product_7e30b/1
  State_id_line_8_9_6201c/1 -> Product_5be2d/2
  State_iq_line_8_9_3d23d/1 -> Product_7e30b/2
  Product_5be2d/1 -> Subtract_f6bd1/1
  Constant_2341.55974180606_2b1bb/1 -> Product_d55c5/1
  Product_7e30b/1 -> Subtract_f6bd1/2
  State_vq_bus_8_ba3ce/1 -> Product_d55c5/2
  Subtract_f6bd1/1 -> Add_051e8/1
  Product_d55c5/1 -> Add_051e8/2
  Constant_2341.55974180606_e9be4/1 -> Product_aa549/1
  Add_051e8/1 -> Subtract_9c8a5/1
  State_vq_bus_9_94e60/1 -> Product_aa549/2
  Product_aa549/1 -> Subtract_9c8a5/2
  Subtract_9c8a5/1 -> Blockout_d_iq_line_8_9_1ac9c/1

== system IEEE9_case/AC_1/d_iq_line_9_4_block ==
  note: d_iq_line_9_4 in IEEE9_case
      | $4435.18962859735\,\mathrm{vq}_{\mathrm{bus},9}-44.3518962859735\,\mathrm{iq}_{\mathrm{line},9,4}-4435.18962859735\,\mathrm{vq}_{\mathrm{bus},4}-376.991118430775\,\mathrm{id}_{\mathrm{line},9,4}$
      | Automatically generated on 2025-11-01 08:51:17 .
  State_id_line_9_4_42230 : Inport
  State_iq_line_9_4_0d177 : Inport  Port=2
  State_vq_bus_4_bde9c : Inport  Port=3
  State_vq_bus_9_ed765 : Inport  Port=4
  Add_f19fd : Sum
  Constant_-376.991118430775_48e7b : Constant  Value=-376.991118430775
  Constant_44.3518962859735_e59a7 : Constant  Value=44.3518962859735
  Constant_4435.18962859735_b062d : Constant  Value=4435.18962859735
  Constant_4435.18962859735_dc698 : Constant  Value=4435.18962859735
  Product_03fbc : Product
  Product_42a6d : Product
  Product_4b89f : Product
  Product_ec21c : Product
  Subtract_477d4 : Sum  Inputs=+-
  Subtract_7665b : Sum  Inputs=+-
  Blockout_d_iq_line_9_4_c7246 : Outport
  wires:
  Constant_-376.991118430775_48e7b/1 -> Product_4b89f/1
  Constant_44.3518962859735_e59a7/1 -> Product_42a6d/1
  State_id_line_9_4_42230/1 -> Product_4b89f/2
  State_iq_line_9_4_0d177/1 -> Product_42a6d/2
  Product_4b89f/1 -> Subtract_7665b/1
  Constant_4435.18962859735_b062d/1 -> Product_03fbc/1
  Product_42a6d/1 -> Subtract_7665b/2
  State_vq_bus_4_bde9c/1 -> Product_03fbc/2
  Subtract_7665b/1 -> Subtract_477d4/1
  Product_03fbc/1 -> Subtract_477d4/2
  Constant_4435.18962859735_dc698/1 -> Product_ec21c/1
  Add_f19fd/1 -> Blockout_d_iq_line_9_4_c7246/1
  State_vq_bus_9_ed765/1 -> Product_ec21c/2
  Subtract_477d4/1 -> Add_f19fd/1
  Product_ec21c/1 -> Add_f19fd/2

== system IEEE9_case/AC_1/d_iq_load_5_block ==
  note: d_iq_load_5 in IEEE9_case
      | $1188.5640696821\,\mathrm{vq}_{\mathrm{bus},5}-1130.97335529233\,\mathrm{iq}_{\mathrm{load},5}-376.991118430775\,\mathrm{id}_{\mathrm{load},5}$
      | Automatically generated on 2025-11-01 08:50:53 .
  State_id_load_5_10f5e : Inport
  State_iq_load_5_7c17a : Inport  Port=2
  State_vq_bus_5_98bbe : Inport  Port=3
  Add_ab403 : Sum
  Constant_-376.991118430775_fe6d5 : Constant  Value=-376.991118430775
  Constant_1130.97335529233_79b00 : Constant  Value=1130.97335529233
  Constant_1188.5640696821_1c3cf : Constant  Value=1188.5640696821
  Product_7b090 : Product
  Product_b06fc : Product
  Product_b127d : Product
  Subtract_510a2 : Sum  Inputs=+-
  Blockout_d_iq_load_5_e7eeb : Outport
  wires:
  Constant_-376.991118430775_fe6d5/1 -> Product_7b090/1
  Product_b06fc/1 -> Subtract_510a2/2
  State_id_load_5_10f5e/1 -> Product_7b090/2
  Constant_1130.97335529233_79b00/1 -> Product_b06fc/1
  Product_7b090/1 -> Subtract_510a2/1
  State_iq_load_5_7c17a/1 -> Product_b06fc/2
  Constant_1188.5640696821_1c3cf/1 -> Product_b127d/1
  State_vq_bus_5_98bbe/1 -> Product_b127d/2
  Subtract_510a2/1 -> Add_ab403/1
  Product_b127d/1 -> Add_ab403/2
  Add_ab403/1 -> Blockout_d_iq_load_5_e7eeb/1

== system IEEE9_case/AC_1/d_iq_load_7_block ==
  note: d_iq_load_7 in IEEE9_case
      | $1244.53892235533\,\mathrm{vq}_{\mathrm{bus},7}-1077.11748123079\,\mathrm{iq}_{\mathrm{load},7}-376.991118430775\,\mathrm{id}_{\mathrm{load},7}$
      | Automatically generated on 2025-11-01 08:50:55 .
  State_id_load_7_95f0d : Inport
  State_iq_load_7_fd2d1 : Inport  Port=2
  State_vq_bus_7_f7a5b : Inport  Port=3
  Add_e3edd : Sum
  Constant_-376.991118430775_008e7 : Constant  Value=-376.991118430775
  Constant_1077.11748123079_6a6e7 : Constant  Value=1077.11748123079
  Constant_1244.53892235533_d18fe : Constant  Value=1244.53892235533
  Product_4a3fe : Product
  Product_8f8bb : Product
  Product_ebe61 : Product
  Subtract_774ce : Sum  Inputs=+-
  Blockout_d_iq_load_7_80412 : Outport
  wires:
  Constant_-376.991118430775_008e7/1 -> Product_4a3fe/1
  Product_8f8bb/1 -> Subtract_774ce/2
  State_id_load_7_95f0d/1 -> Product_4a3fe/2
  Constant_1077.11748123079_6a6e7/1 -> Product_8f8bb/1
  Product_4a3fe/1 -> Subtract_774ce/1
  State_iq_load_7_fd2d1/1 -> Product_8f8bb/2
  Constant_1244.53892235533_d18fe/1 -> Product_ebe61/1
  State_vq_bus_7_f7a5b/1 -> Product_ebe61/2
  Subtract_774ce/1 -> Add_e3edd/1
  Product_ebe61/1 -> Add_e3edd/2
  Add_e3edd/1 -> Blockout_d_iq_load_7_80412/1

== system IEEE9_case/AC_1/d_iq_load_9_block ==
  note: d_iq_load_9 in IEEE9_case
      | $1490.22474585066\,\mathrm{vq}_{\mathrm{bus},9}-942.477796076938\,\mathrm{iq}_{\mathrm{load},9}-376.991118430775\,\mathrm{id}_{\mathrm{load},9}$
      | Automatically generated on 2025-11-01 08:50:57 .
  State_id_load_9_c133f : Inport
  State_iq_load_9_0ed41 : Inport  Port=2
  State_vq_bus_9_4444e : Inport  Port=3
  Add_6c922 : Sum
  Constant_-376.991118430775_240d3 : Constant  Value=-376.991118430775
  Constant_1490.22474585066_95f86 : Constant  Value=1490.22474585066
  Constant_942.477796076938_cf3c0 : Constant  Value=942.477796076938
  Product_11482 : Product
  Product_1ab32 : Product
  Product_efc41 : Product
  Subtract_3b3d5 : Sum  Inputs=+-
  Blockout_d_iq_load_9_bcf8f : Outport
  wires:
  Constant_-376.991118430775_240d3/1 -> Product_efc41/1
  Product_11482/1 -> Subtract_3b3d5/2
  State_id_load_9_c133f/1 -> Product_efc41/2
  Add_6c922/1 -> Blockout_d_iq_load_9_bcf8f/1
  Constant_942.477796076938_cf3c0/1 -> Product_11482/1
  Product_1ab32/1 -> Add_6c922/2
  Product_efc41/1 -> Subtract_3b3d5/1
  State_iq_load_9_0ed41/1 -> Product_11482/2
  Constant_1490.22474585066_95f86/1 -> Product_1ab32/1
  State_vq_bus_9_4444e/1 -> Product_1ab32/2
  Subtract_3b3d5/1 -> Add_6c922/1

== system IEEE9_case/AC_1/d_vd_bus_1_block ==
  note: d_vd_bus_1 in IEEE9_case
      | $37699111.8430775\,\mathrm{id}_{\mathrm{bus},1}+376.991118430775\,\mathrm{vq}_{\mathrm{bus},1}$
      | Automatically generated on 2025-11-01 08:50:38 .
  Alge_id_bus_1_80866 : Inport
  State_vq_bus_1_61947 : Inport  Port=2
  Add_66d16 : Sum
  Constant_376.991118430775_5fbc6 : Constant  Value=376.991118430775
  Constant_37699111.8430775_19751 : Constant  Value=37699111.8430775
  Product_d83c8 : Product
  Product_dd5f9 : Product
  Blockout_d_vd_bus_1_137dc : Outport
  wires:
  Constant_37699111.8430775_19751/1 -> Product_dd5f9/1
  Product_d83c8/1 -> Add_66d16/2
  Alge_id_bus_1_80866/1 -> Product_dd5f9/2
  Constant_376.991118430775_5fbc6/1 -> Product_d83c8/1
  State_vq_bus_1_61947/1 -> Product_d83c8/2
  Add_66d16/1 -> Blockout_d_vd_bus_1_137dc/1
  Product_dd5f9/1 -> Add_66d16/1

== system IEEE9_case/AC_1/d_vd_bus_2_block ==
  note: d_vd_bus_2 in IEEE9_case
      | $37699111.8430775\,\mathrm{id}_{\mathrm{bus},2}+376.991118430775\,\mathrm{vq}_{\mathrm{bus},2}$
      | Automatically generated on 2025-11-01 08:50:39 .
  Alge_id_bus_2_c2beb : Inport
  State_vq_bus_2_66edc : Inport  Port=2
  Add_d64a1 : Sum
  Constant_376.991118430775_ec58b : Constant  Value=376.991118430775
  Constant_37699111.8430775_6c712 : Constant  Value=37699111.8430775
  Product_bc2ef : Product
  Product_ec6d3 : Product
  Blockout_d_vd_bus_2_9f603 : Outport
  wires:
  Constant_37699111.8430775_6c712/1 -> Product_bc2ef/1
  Product_ec6d3/1 -> Add_d64a1/2
  Alge_id_bus_2_c2beb/1 -> Product_bc2ef/2
  Constant_376.991118430775_ec58b/1 -> Product_ec6d3/1
  Product_bc2ef/1 -> Add_d64a1/1
  State_vq_bus_2_66edc/1 -> Product_ec6d3/2
  Add_d64a1/1 -> Blockout_d_vd_bus_2_9f603/1

== system IEEE9_case/AC_1/d_vd_bus_3_block ==
  note: d_vd_bus_3 in IEEE9_case
      | $37699111.8430775\,\mathrm{id}_{\mathrm{bus},3}+376.991118430775\,\mathrm{vq}_{\mathrm{bus},3}$
      | Automatically generated on 2025-11-01 08:50:41 .
  Alge_id_bus_3_a6e23 : Inport
  State_vq_bus_3_26672 : Inport  Port=2
  Add_a915a : Sum
  Constant_376.991118430775_14364 : Constant  Value=376.991118430775
  Constant_37699111.8430775_c1364 : Constant  Value=37699111.8430775
  Product_0f62a : Product
  Product_8f490 : Product
  Blockout_d_vd_bus_3_85bef : Outport
  wires:
  Constant_37699111.8430775_c1364/1 -> Product_8f490/1
  Product_0f62a/1 -> Add_a915a/2
  Alge_id_bus_3_a6e23/1 -> Product_8f490/2
  Constant_376.991118430775_14364/1 -> Product_0f62a/1
  Product_8f490/1 -> Add_a915a/1
  State_vq_bus_3_26672/1 -> Product_0f62a/2
  Add_a915a/1 -> Blockout_d_vd_bus_3_85bef/1

== system IEEE9_case/AC_1/d_vd_bus_4_block ==
  note: d_vd_bus_4 in IEEE9_case
      | $2257.43184689087\,\mathrm{id}_{\mathrm{bus},4}+376.991118430775\,\mathrm{vq}_{\mathrm{bus},4}$
      | Automatically generated on 2025-11-01 08:50:42 .
  Alge_id_bus_4_4fdbe : Inport
  State_vq_bus_4_0d84f : Inport  Port=2
  Add_725a6 : Sum
  Constant_2257.43184689087_e568f : Constant  Value=2257.43184689087
  Constant_376.991118430775_e0f14 : Constant  Value=376.991118430775
  Product_4379a : Product
  Product_573dc : Product
  Blockout_d_vd_bus_4_55aab : Outport
  wires:
  Constant_2257.43184689087_e568f/1 -> Product_4379a/1
  Product_573dc/1 -> Add_725a6/2
  Alge_id_bus_4_4fdbe/1 -> Product_4379a/2
  Constant_376.991118430775_e0f14/1 -> Product_573dc/1
  Product_4379a/1 -> Add_725a6/1
  State_vq_bus_4_0d84f/1 -> Product_573dc/2
  Add_725a6/1 -> Blockout_d_vd_bus_4_55aab/1

== system IEEE9_case/AC_1/d_vd_bus_5_block ==
  note: d_vd_bus_5 in IEEE9_case
      | $1461.2058853906\,\mathrm{id}_{\mathrm{bus},5}+376.991118430775\,\mathrm{vq}_{\mathrm{bus},5}$
      | Automatically generated on 2025-11-01 08:50:44 .
  Alge_id_bus_5_5b93e : Inport
  State_vq_bus_5_adcb7 : Inport  Port=2
  Add_b3133 : Sum
  Constant_1461.2058853906_89b23 : Constant  Value=1461.2058853906
  Constant_376.991118430775_d57da : Constant  Value=376.991118430775
  Product_08f49 : Product
  Product_a7e25 : Product
  Blockout_d_vd_bus_5_d9166 : Outport
  wires:
  Constant_1461.2058853906_89b23/1 -> Product_a7e25/1
  Product_08f49/1 -> Add_b3133/2
  Alge_id_bus_5_5b93e/1 -> Product_a7e25/2
  Constant_376.991118430775_d57da/1 -> Product_08f49/1
  Product_a7e25/1 -> Add_b3133/1
  State_vq_bus_5_adcb7/1 -> Product_08f49/2
  Add_b3133/1 -> Blockout_d_vd_bus_5_d9166/1

== system IEEE9_case/AC_1/d_vd_bus_6_block ==
  note: d_vd_bus_6 in IEEE9_case
      | $1329.77466818616\,\mathrm{id}_{\mathrm{bus},6}+376.991118430775\,\mathrm{vq}_{\mathrm{bus},6}$
      | Automatically generated on 2025-11-01 08:50:45 .
  Alge_id_bus_6_7ffa8 : Inport
  State_vq_bus_6_8f435 : Inport  Port=2
  Add_cd9b4 : Sum
  Constant_1329.77466818616_e3ea2 : Constant  Value=1329.77466818616
  Constant_376.991118430775_94581 : Constant  Value=376.991118430775
  Product_eeffa : Product
  Product_f299d : Product
  Blockout_d_vd_bus_6_cbe78 : Outport
  wires:
  Constant_1329.77466818616_e3ea2/1 -> Product_f299d/1
  Product_eeffa/1 -> Add_cd9b4/2
  Alge_id_bus_6_7ffa8/1 -> Product_f299d/2
  Constant_376.991118430775_94581/1 -> Product_eeffa/1
  Product_f299d/1 -> Add_cd9b4/1
  State_vq_bus_6_8f435/1 -> Product_eeffa/2
  Add_cd9b4/1 -> Blockout_d_vd_bus_6_cbe78/1

== system IEEE9_case/AC_1/d_vd_bus_7_block ==
  note: d_vd_bus_7 in IEEE9_case
      | $2106.09563369148\,\mathrm{id}_{\mathrm{bus},7}+376.991118430775\,\mathrm{vq}_{\mathrm{bus},7}$
      | Automatically generated on 2025-11-01 08:50:47 .
  Alge_id_bus_7_08ef0 : Inport
  State_vq_bus_7_85f46 : Inport  Port=2
  Add_eec8b : Sum
  Constant_2106.09563369148_5e71a : Constant  Value=2106.09563369148
  Constant_376.991118430775_c2493 : Constant  Value=376.991118430775
  Product_122bb : Product
  Product_b5771 : Product
  Blockout_d_vd_bus_7_6d513 : Outport
  wires:
  Constant_2106.09563369148_5e71a/1 -> Product_b5771/1
  Product_122bb/1 -> Add_eec8b/2
  Alge_id_bus_7_08ef0/1 -> Product_b5771/2
  Constant_376.991118430775_c2493/1 -> Product_122bb/1
  Product_b5771/1 -> Add_eec8b/1
  State_vq_bus_7_85f46/1 -> Product_122bb/2
  Add_eec8b/1 -> Blockout_d_vd_bus_7_6d513/1

== system IEEE9_case/AC_1/d_vd_bus_8_block ==
  note: d_vd_bus_8 in IEEE9_case
      | $1657.10381727813\,\mathrm{id}_{\mathrm{bus},8}+376.991118430775\,\mathrm{vq}_{\mathrm{bus},8}$
      | Automatically generated on 2025-11-01 08:50:49 .
  Alge_id_bus_8_85559 : Inport
  State_vq_bus_8_ca02b : Inport  Port=2
  Add_fcda8 : Sum
  Constant_1657.10381727813_b8fed : Constant  Value=1657.10381727813
  Constant_376.991118430775_342ad : Constant  Value=376.991118430775
  Product_8dcd5 : Product
  Product_cd047 : Product
  Blockout_d_vd_bus_8_71a28 : Outport
  wires:
  Constant_1657.10381727813_b8fed/1 -> Product_cd047/1
  Product_8dcd5/1 -> Add_fcda8/2
  Alge_id_bus_8_85559/1 -> Product_cd047/2
  Constant_376.991118430775_342ad/1 -> Product_8dcd5/1
  Product_cd047/1 -> Add_fcda8/1
  State_vq_bus_8_ca02b/1 -> Product_8dcd5/2
  Add_fcda8/1 -> Blockout_d_vd_bus_8_71a28/1

== system IEEE9_case/AC_1/d_vd_bus_9_block ==
  note: d_vd_bus_9 in IEEE9_case
      | $1564.27849971276\,\mathrm{id}_{\mathrm{bus},9}+376.991118430775\,\mathrm{vq}_{\mathrm{bus},9}$
      | Automatically generated on 2025-11-01 08:50:50 .
  Alge_id_bus_9_44435 : Inport
  State_vq_bus_9_fb0a9 : Inport  Port=2
  Add_010fa : Sum
  Constant_1564.27849971276_0b35c : Constant  Value=1564.27849971276
  Constant_376.991118430775_f67ee : Constant  Value=376.991118430775
  Product_052e8 : Product
  Product_fb0dd : Product
  Blockout_d_vd_bus_9_9824e : Outport
  wires:
  Constant_1564.27849971276_0b35c/1 -> Product_052e8/1
  Product_fb0dd/1 -> Add_010fa/2
  Alge_id_bus_9_44435/1 -> Product_052e8/2
  Constant_376.991118430775_f67ee/1 -> Product_fb0dd/1
  Product_052e8/1 -> Add_010fa/1
  State_vq_bus_9_fb0a9/1 -> Product_fb0dd/2
  Add_010fa/1 -> Blockout_d_vd_bus_9_9824e/1

== system IEEE9_case/AC_1/d_vq_bus_1_block ==
  note: d_vq_bus_1 in IEEE9_case
      | $37699111.8430775\,\mathrm{iq}_{\mathrm{bus},1}-376.991118430775\,\mathrm{vd}_{\mathrm{bus},1}$
      | Automatically generated on 2025-11-01 08:50:38 .
  Alge_iq_bus_1_fd912 : Inport
  State_vd_bus_1_380c1 : Inport  Port=2
  Constant_376.991118430775_4e157 : Constant  Value=376.991118430775
  Constant_37699111.8430775_43b63 : Constant  Value=37699111.8430775
  Product_57225 : Product
  Product_9a8f4 : Product
  Subtract_db6a7 : Sum  Inputs=+-
  Blockout_d_vq_bus_1_1e70c : Outport
  wires:
  Constant_37699111.8430775_43b63/1 -> Product_57225/1
  Constant_376.991118430775_4e157/1 -> Product_9a8f4/1
  Alge_iq_bus_1_fd912/1 -> Product_57225/2
  State_vd_bus_1_380c1/1 -> Product_9a8f4/2
  Product_57225/1 -> Subtract_db6a7/1
  Product_9a8f4/1 -> Subtract_db6a7/2
  Subtract_db6a7/1 -> Blockout_d_vq_bus_1_1e70c/1

== system IEEE9_case/AC_1/d_vq_bus_2_block ==
  note: d_vq_bus_2 in IEEE9_case
      | $37699111.8430775\,\mathrm{iq}_{\mathrm{bus},2}-376.991118430775\,\mathrm{vd}_{\mathrm{bus},2}$
      | Automatically generated on 2025-11-01 08:50:40 .
  Alge_iq_bus_2_afa01 : Inport
  State_vd_bus_2_6eee7 : Inport  Port=2
  Constant_376.991118430775_c60f8 : Constant  Value=376.991118430775
  Constant_37699111.8430775_1ddb9 : Constant  Value=37699111.8430775
  Product_60f7c : Product
  Product_b93af : Product
  Subtract_528e0 : Sum  Inputs=+-
  Blockout_d_vq_bus_2_09653 : Outport
  wires:
  Constant_37699111.8430775_1ddb9/1 -> Product_60f7c/1
  Constant_376.991118430775_c60f8/1 -> Product_b93af/1
  Alge_iq_bus_2_afa01/1 -> Product_60f7c/2
  State_vd_bus_2_6eee7/1 -> Product_b93af/2
  Product_60f7c/1 -> Subtract_528e0/1
  Product_b93af/1 -> Subtract_528e0/2
  Subtract_528e0/1 -> Blockout_d_vq_bus_2_09653/1

== system IEEE9_case/AC_1/d_vq_bus_3_block ==
  note: d_vq_bus_3 in IEEE9_case
      | $37699111.8430775\,\mathrm{iq}_{\mathrm{bus},3}-376.991118430775\,\mathrm{vd}_{\mathrm{bus},3}$
      | Automatically generated on 2025-11-01 08:50:42 .
  Alge_iq_bus_3_cccc7 : Inport
  State_vd_bus_3_d37be : Inport  Port=2
  Constant_376.991118430775_46092 : Constant  Value=376.991118430775
  Constant_37699111.8430775_c9e12 : Constant  Value=37699111.8430775
  Product_c35c0 : Product
  Product_eb1f9 : Product
  Subtract_eb0bd : Sum  Inputs=+-
  Blockout_d_vq_bus_3_e2948 : Outport
  wires:
  Constant_37699111.8430775_c9e12/1 -> Product_c35c0/1
  Constant_376.991118430775_46092/1 -> Product_eb1f9/1
  Alge_iq_bus_3_cccc7/1 -> Product_c35c0/2
  State_vd_bus_3_d37be/1 -> Product_eb1f9/2
  Product_c35c0/1 -> Subtract_eb0bd/1
  Product_eb1f9/1 -> Subtract_eb0bd/2
  Subtract_eb0bd/1 -> Blockout_d_vq_bus_3_e2948/1
